simulink library "SystemPulse"  (Simulink 8.2)
settings: Solver=ode45  StartTime=0.0  StopTime=10.0  RelTol=1e-3
settings Model: Creator=lena.frank  LastModifiedBy=drhf

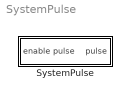
== system SystemPulse ==
  SystemPulse : Subsystem  mask(system pulse){enable_flag=on, datecheck=off, date=[2 10 10 36 15], period=5, pulsewidth=2}
      mask prompts: enable_flag "Wait for enabling pulse"; datecheck "Wait for start date"; date "start date [month day hour minute second]"; period "period [s]"; pulsewidth "pulse width [s]"
      mask help:
      | This block generates a discrete pulse of 0 and 1, but this pulse depends on the system time, not the simulation time.
      | If the date flag is set, the function starts pulsing only when the system date reaches the specified date. Otherwise the output is 0.
      | If the enable flag is set, the function waits, until the enabling pulse once rise from 0 to 1. Afterwards the pulsing is started. Before pulsing the output will be 0.
      mask Help: web(fullfile(path_carnot('help'),'SystemPulse.html'),'-helpbrowser')

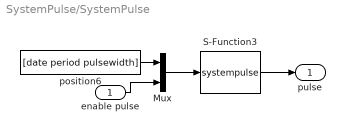
== system SystemPulse/SystemPulse ==
  enable pulse : Inport
  Mux : Mux  Inputs=2
  S-Function3 : S-Function  FunctionName=systempulse  Parameters=datecheck enable_flag  EnableBusSupport=off
  position6 : Constant  Value=[date period pulsewidth]
  pulse : Outport
  wires:
  position6/1 -> Mux/1
  S-Function3/1 -> pulse/1
  enable pulse/1 -> Mux/2
  Mux/1 -> S-Function3/1
